simulink model "sldemo_mdlref_basic"  (R2025b)
settings: Solver=FixedStepDiscrete  StartTime=0.0  StopTime=10.0  FixedStep=0.1  RelTol=1e-3
InitFcn:
  | warning('off','Simulink:Logging:DatasetRTWGenRootOutputNotSupported');
  | warning('off','Simulink:Logging:DatasetRTWGenStateNotSupported');
StartFcn:
  | warning('off','Simulink:Logging:DatasetRTWGenRootOutputNotSupported');
  | warning('off','Simulink:Logging:DatasetRTWGenStateNotSupported');
StopFcn:
  | warning('on','Simulink:Logging:DatasetRTWGenRootOutputNotSupported');
  | warning('on','Simulink:Logging:DatasetRTWGenStateNotSupported');
CloseFcn:
  | warning('on','Simulink:Logging:DatasetRTWGenRootOutputNotSupported');
  | warning('on','Simulink:Logging:DatasetRTWGenStateNotSupported');
PauseFcn:
  | warning('on','Simulink:Logging:DatasetRTWGenRootOutputNotSupported');
  | warning('on','Simulink:Logging:DatasetRTWGenStateNotSupported');
settings Model: ModifiedByFormat=The MathWorks Inc.  ExtModeAutoUpdateStatusClock=off  Creator=The MathWorks, Inc.  LastModifiedBy=The MathWorks Inc.
settings SolverCC: AlgebraicLoopSolver=TrustRegion
settings DataIOCC: LimitDataPoints=on  SaveFinalState=on  SaveState=on  SignalLoggingName=logsOut
settings OptimizationCC: DefaultParameterBehavior=Inlined  InlineInvariantSignals=on  ExpressionDepthLimit=2147483647.0  InitFltsAndDblsToZero=on  LifeSpan=inf
settings DebuggingCC: SaveWithParameterizedLinksMsg=none  CheckExecutionContextPreStartOutputMsg=on  MultiTaskDSMMsg=warning  MultiTaskCondExecSysMsg=none  SigSpecEnsureSampleTimeMsg=none  FcnCallInpInsideContextMsg=warning  UnconnectedInputMsg=warning  UnconnectedOutputMsg=warning  UnconnectedLineMsg=warning  AllowSymbolicDim=off  StateNameClashWarn=warning  StrictBusMsg=ErrorOnBusTreatedAsVector  SFUnexpectedBacktrackingDiag=warning  SFNoUnconditionalDefaultTransitionDiag=warning  SFExecutionAtInitializationDiag=none  ArithmeticOperatorsInVariantConditions=warning
settings HardwareCC: ProdBitPerPointer=32.0  ProdBitPerSizeT=32.0  ProdBitPerPtrDiffT=32.0  ProdLargestAtomicFloat=None  ProdIntDivRoundTo=Undefined  ProdEndianess=Unspecified  ProdWordSize=32.0  ProdHWDeviceType=32-bit Generic  TargetHWDeviceType=32-bit Generic
settings ModelReferenceCC: UpdateModelReferenceTargets=IfOutOfDate  EnableRefExpFcnMdlSchedulingChecks=on  CheckModelReferenceTargetMessage=none  PropagateSignalLabelsOutOfModel=off
settings SFSimCC: SimUseLocalCustomCode=off  CustomCodeUndefinedFunction=UseInterfaceOnly
settings RTWCC: GenerateReport=on  RTWUseLocalCustomCode=off  LaunchReport=on  GPUComputeCapability=3.5  DLArmComputeVersion=19.05
settings CodeAppCC: MaxIdLength=100.0  StateflowObjectComments=on
settings GRTTargetCC: TargetFcnLib=ansi_tfl_tmw.mat  TargetLangStandard=C89/C90 (ANSI)  CombineOutputUpdateFcns=off  GRTInterface=on
settings ConfigComp: CovMetricSettings=dw  CovSaveCumulativeToWorkspaceVar=on  CovSaveSingleToWorkspaceVar=on  CovExternalEMLEnable=off  CovSFcnEnable=off

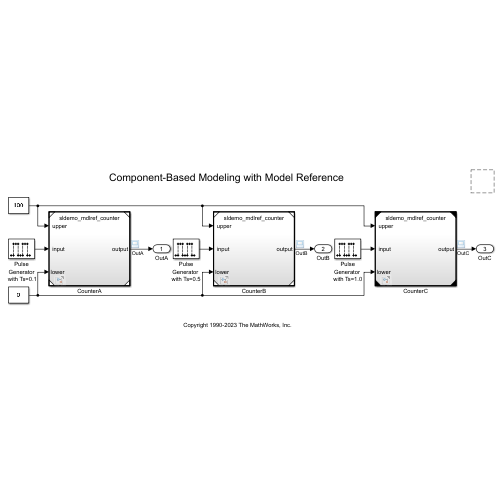
[thumbnail: Simulink's stored preview of the top-level diagram]
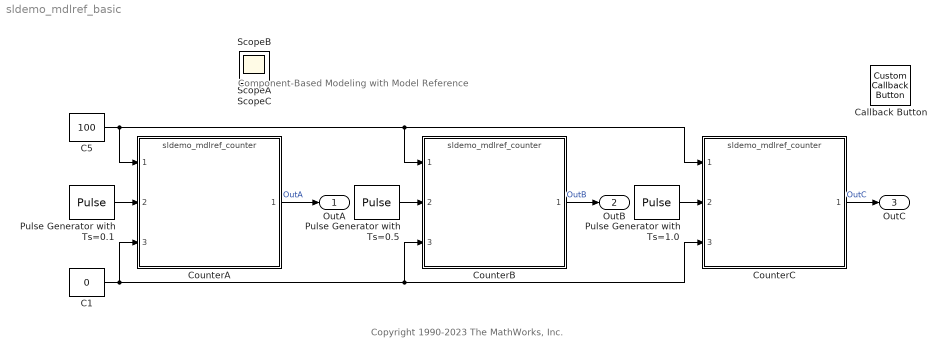
== system sldemo_mdlref_basic ==
  note: Component-Based Modeling with Model Reference
  note: Copyright 1990-2023 The MathWorks, Inc.
  C1 : Constant  Value=0
  C5 : Constant  Value=100
  Callback Button : CustomCallbackButton  Configuration="{\"components\":[{\"name\":\"BackgroundImageComponent\",\"settings\":{\"image\":{\"size\":[0,0],\"src\":\"default\",\"srcOrientation\":\"Right\"},\"position\":[0,0,1,1]}},{\"name\":\"ButtonStateComponent\",\"settings\":{\"buttonType\":\"momentary\",\"clickFcn\":\"showExample('simulink\\/ExamineMultipleReferencedModelInstancesExample')\",\"onValue\":1,\"position\":[0,0,1,1],\"pressDelay\":\"500\",\"pressFcn\":\"\",\"repeatInterval\":\"0\",\"states\":[{\"horizontalAlignment\":\"center\",\"image\":{\"position\":[0,0,1,1],\"size\":[1,1],\"src\":\"default\",\"srcOrientation\":\"Right\"},\"label\":{\"color\":[0.01176470588,0.01176470588,0.01176470588,1],\"icon\":{\"size\":[0,0],\"src\":\"default\",\"srcOrientation\":\"Right\"},\"iconPlacement\":\"left\",\"opacity\":1,\"show\":true,\"text\":{\"content\":\"?\",\"font\":\"Helvetica\",\"fontSize\":12}},\"labelOffset\":[0,0],\"verticalAlignment\":\"middle\"},{\"horizontalAlignment\":\"center\",\"image\":{\"position\":[0,0,1,1],\"size\":[1,1],\"src\":\"default\",\"srcOrientation\":\"Right\"},\"label\":{\"color\":[0.01176470588,0.01176470588,0.01176470588,1],\"icon\":{\"size\":[0,0],\"src\":\"default\",\"srcOrientation\":\"Right\"},\"iconPlacement\":\"left\",\"opacity\":1,\"show\":true,\"text\":{\"content\":\"?\",\"font\":\"Helvetica\",\"fontSize\":12}},\"labelOffset\":[0,0],\"verticalAlignment\":\"middle\"},{\"horizontalAlignment\":\"center\",\"image\":{\"position\":[0,0,1,1],\"size\":[1,1],\"src\":\"default\",\"srcOrientation\":\"Right\"},\"label\":{\"color\":[0.01176470588,0.01176470588,0.01176470588,1],\"icon\":{\"size\":[0,0],\"src\":\"default\",\"srcOrientation\":\"Right\"},\"iconPlacement\":\"left\",\"opacity\":1,\"show\":true,\"text\":{\"content\":\"?\",\"font\":\"Helvetica\",\"fontSize\":12}},\"labelOffset\":[0,0],\"verticalAlignment\":\"middle\"},{\"horizontalAlignment\":\"center\",\"image\":{\"position\":[0,0,1,1],\"size\":[1,1],\"src\":\"default\",\"srcOrientation\":\"Right\"},\"label\":{\"color\":[0.01176470588,0.01176470588,0.01176470588,1],\"icon\":{\"size\":[0,0],\"src\":\"default\",\"srcOrientation\":\"Right\"},\"iconPlacement\":\"left\",\"opacity\":1,\"show\":true,\"text\":{\"content\":\"?\",\"font\":\"Helvetica\",\"fontSize\":12}},\"labelOffset\":[0,0],\"verticalAlignment\":\"middle\"}]}},{\"name\":\"ForegroundImageComponent\",\"settings\":{\"image\":{\"size\":[0,0],\"src\":\"default\",\"srcOrientation\":\"Right\"},\"isForeground\":1,\"position\":[0,0,1,1]}}],\"settings\":{\"BindingType\":\"standalone\",\"backgroundColor\":[244,244,244,1],\"backgroundOffset\":0.2,\"backgroundOpacity\":1,\"fixedAspectRatio\":\"off\",\"foregroundColor\":[0.01176470588,0.01176470588,0.01176470588,1],\"migratedFromLegacy\":true,\"useBackgroundColor\":true,\"variant\":\"callback\",\"version\":\"R2023a\"},\"type\":\"Button\"}"  CustomBackgroundColor="{\"color\":[0.9568627451,0.9568627451,0.9568627451],\"show\":true}"
  CounterA : ModelReference  ModelNameDialog=sldemo_mdlref_counter  SimulationMode=Normal  ModelReferenceVersion=11.0
  CounterB : ModelReference  ModelNameDialog=sldemo_mdlref_counter  SimulationMode=Normal  ModelReferenceVersion=11.0
  CounterC : ModelReference  ModelNameDialog=sldemo_mdlref_counter  ModelReferenceVersion=11.0
  Pulse Generator with Ts=0.1 : DiscretePulseGenerator  SampleTime=0.1  VectorParams1D=off
  Pulse Generator with Ts=0.5 : DiscretePulseGenerator  SampleTime=0.5
  Pulse Generator with Ts=1.0 : DiscretePulseGenerator  SampleTime=1.0
  OutA : Outport  VectorParamsAs1DForOutWhenUnconnected=off
  OutB : Outport  Port=2  VectorParamsAs1DForOutWhenUnconnected=off
  OutC : Outport  Port=3  VectorParamsAs1DForOutWhenUnconnected=off
  ScopeA : Scope
      settings: TimeSpan=10  ActiveDisplayYMinimum=0  ActiveDisplayYMaximum=100
  ScopeB : Scope
      settings: TimeSpan=10  ActiveDisplayYMinimum=0  ActiveDisplayYMaximum=25
  ScopeC : Scope
      settings: TimeSpan=10  ActiveDisplayYMinimum=0  ActiveDisplayYMaximum=15  DataLoggingVariableName=ScopeData2
  wires:
  CounterB/1 -> OutB/1  "OutB"
  CounterA/1 -> OutA/1  "OutA"
  CounterC/1 -> OutC/1  "OutC"
  Pulse Generator with Ts=0.1/1 -> CounterA/2
  Pulse Generator with Ts=0.5/1 -> CounterB/2
  Pulse Generator with Ts=1.0/1 -> CounterC/2
  C1/1 -> CounterA/3, CounterB/3, CounterC/3
  C5/1 -> CounterA/1, CounterB/1, CounterC/1
